simulink model "decibel_baseline"  (R2018a)
settings: Solver=VariableStepAuto  StartTime=0.0  StopTime=10e-3  RelTol=1e-3
libraries: simulink x1
settings Model: Creator=alex8  LastModifiedBy=alex8

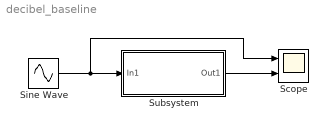
== system decibel_baseline ==
  Scope : Scope  NumInputPorts=2
  Sine Wave : Sin  Frequency=2*pi*1e3  SampleTime=0
  Subsystem : Subsystem
  wires:
  Sine Wave/1 -> Scope/1, Subsystem/1(In1)
  Subsystem/1(Out1) -> Scope/2

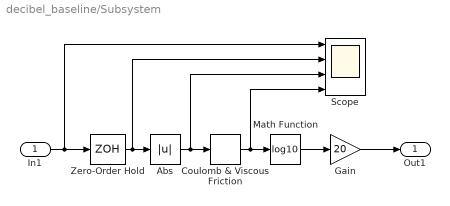
== system decibel_baseline/Subsystem ==
  In1 : Inport
  Abs : Abs
  Coulomb & Viscous Friction : simulink/Discontinuities/Coulomb & Viscous Friction  offset=1e-4  gain=1
      settings: SourceProductName=Simulink
  Gain : Gain  Gain=20
  Math Function : Math  Operator=log10  SaturateOnIntegerOverflow=on
  Scope : Scope  NumInputPorts=4
  Zero-Order Hold : ZeroOrderHold  SampleTime=1/44100
  Out1 : Outport
  wires:
  In1/1 -> Scope/1, Zero-Order Hold/1
  Math Function/1 -> Gain/1
  Gain/1 -> Out1/1
  Zero-Order Hold/1 -> Scope/2, Abs/1
  Abs/1 -> Scope/3, Coulomb & Viscous Friction/1
  Coulomb & Viscous Friction/1 -> Scope/4, Math Function/1
